simulink model "CoTS_MechDem"  (R2016b)
settings: configuration reference "CodeGenConfigSet" (kept outside this file)
values from neighbouring files (symbols this model uses):
  TS_nMax_C = Calibration.Parameter    [init_CoTS_MechDem.m]    (also in init_CoTS_MechDem_SIL.m = Simulink.Parameter)
  TS_nMin_C = Calibration.Parameter    [init_CoTS_MechDem.m]    (also in init_CoTS_MechDem_SIL.m = Simulink.Parameter)
  TS_trqDesAcs_C = Calibration.Parameter    [init_CoTS_MechDem.m]    (also in init_CoTS_MechDem_SIL.m = Simulink.Parameter)
  TS_trqResvAcs_C = Calibration.Parameter    [init_CoTS_MechDem.m]    (also in init_CoTS_MechDem_SIL.m = Simulink.Parameter)
settings Model: Creator=Wollf  LastModifiedBy=xinchangran
settings ConfigSetRef: SourceLocation=Base Workspace

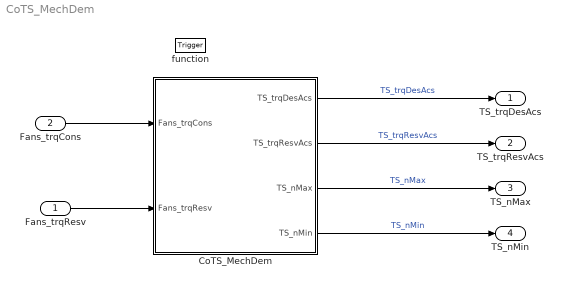
== system CoTS_MechDem ==
  Fans_trqResv : Inport  Tag=Nm  Description=Torque reserve for cooling fan  OutMin=-3000  OutMax=3000  OutDataTypeStr=Trq_Nm
  Fans_trqCons : Inport  Tag=Nm  Description=Torque consumed by Fan  Port=2  OutMin=-3000  OutMax=3000  OutDataTypeStr=Trq_Nm
  function : TriggerPort  TriggerType=function-call  VariantControl=Variant
  CoTS_MechDem : Subsystem
  TS_trqDesAcs : Outport  Tag=Nm  Description=Desired Torque demand of the thermal system  OutMin=-3000  OutMax=3276.7  OutDataTypeStr=Trq_Nm
  TS_trqResvAcs : Outport  Tag=Nm  Description=Torque reserve of the thermal system  Port=2  OutMin=-3000  OutMax=3276.7  OutDataTypeStr=Trq_Nm
  TS_nMax : Outport  Tag=rpm  Description=Highest engine speed requested by the thermal system  Port=3  OutMin=-12000  OutMax=12000  OutDataTypeStr=EngSpeed_rpm
  TS_nMin : Outport  Tag=rpm  Description=Lowest engine speed requested by the thermal system  Port=4  OutMin=-12000  OutMax=12000  OutDataTypeStr=EngSpeed_rpm
  wires:
  Fans_trqCons/1 -> CoTS_MechDem/1(Fans_trqCons)
  Fans_trqResv/1 -> CoTS_MechDem/2(Fans_trqResv)
  CoTS_MechDem/1(TS_trqDesAcs) -> TS_trqDesAcs/1  "TS_trqDesAcs"
  CoTS_MechDem/2(TS_trqResvAcs) -> TS_trqResvAcs/1  "TS_trqResvAcs"
  CoTS_MechDem/3(TS_nMax) -> TS_nMax/1  "TS_nMax"
  CoTS_MechDem/4(TS_nMin) -> TS_nMin/1  "TS_nMin"

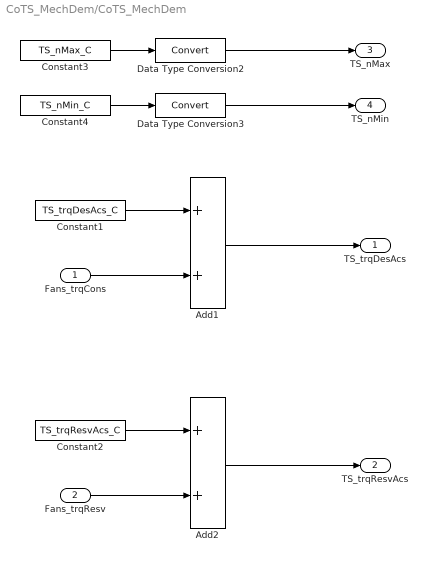
== system CoTS_MechDem/CoTS_MechDem ==
  Fans_trqCons : Inport
  Fans_trqResv : Inport  Port=2
  Add1 : Sum  SaturateOnIntegerOverflow=on  InputSameDT=on
  Add2 : Sum  SaturateOnIntegerOverflow=on  InputSameDT=on
  Constant1 : Constant  Value=TS_trqDesAcs_C
  Constant2 : Constant  Value=TS_trqResvAcs_C
  Constant3 : Constant  Value=TS_nMax_C
  Constant4 : Constant  Value=TS_nMin_C
  Data Type Conversion2 : DataTypeConversion
  Data Type Conversion3 : DataTypeConversion
  TS_trqDesAcs : Outport  Tag=Nm  Description=Desired Torque demand of the thermal system  OutMin=-3000  OutMax=3276.7  OutDataTypeStr=Trq_Nm
  TS_trqResvAcs : Outport  Tag=Nm  Description=Torque reserve of the thermal system  Port=2  OutMin=-3000  OutMax=3276.7  OutDataTypeStr=Trq_Nm
  TS_nMax : Outport  Tag=rpm  Description=Highest engine speed requested by the thermal system  Port=3  OutMin=-12000  OutMax=12000  OutDataTypeStr=EngSpeed_rpm
  TS_nMin : Outport  Tag=rpm  Description=Lowest engine speed requested by the thermal system  Port=4  OutMin=-12000  OutMax=12000  OutDataTypeStr=EngSpeed_rpm
  wires:
  Fans_trqCons/1 -> Add1/2
  Constant2/1 -> Add2/1
  Data Type Conversion3/1 -> TS_nMin/1
  Constant4/1 -> Data Type Conversion3/1
  Add1/1 -> TS_trqDesAcs/1
  Add2/1 -> TS_trqResvAcs/1
  Data Type Conversion2/1 -> TS_nMax/1
  Constant1/1 -> Add1/1
  Constant3/1 -> Data Type Conversion2/1
  Fans_trqResv/1 -> Add2/2
